simulink model "SingleEcho"  (R2024a)
settings: Solver=VariableStepAuto  StartTime=0  StopTime=inf  RelTol=1e-3
libraries: dspsrcs4 x2, audiosources x1, dspsnks4 x1
settings Model: Creator=johannesarizie  LastModifiedBy=johannesarizie

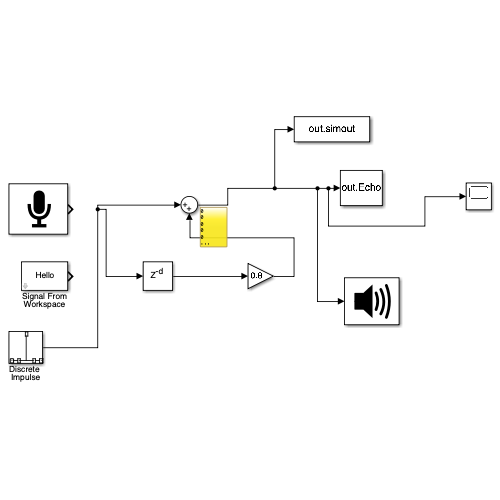
[thumbnail: Simulink's stored preview of the top-level diagram]
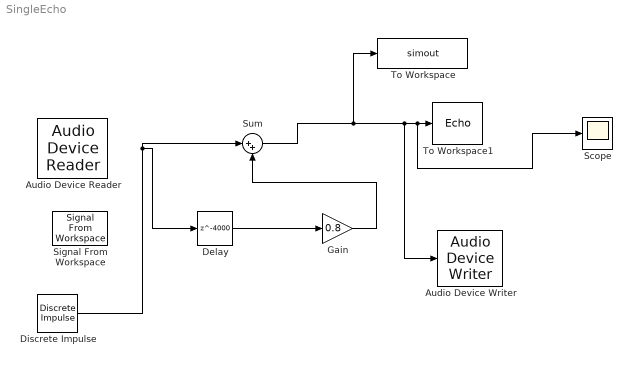
== system SingleEcho ==
  Audio Device Reader : audiosources/Audio Device Reader  Driver=CoreAudio  Device=Default  SampleRate=44100  NumChannels=1  SamplesPerFrame=1024  BitDepth=16-bit integer  NumBuffers=10  DefaultInputChannelMapping=on  InputChannelMapping=1:2  OutputNumOverrunSamples=off  OutputDataType=double  DriverIdx=5  DeviceWarnFlag=''
  Audio Device Writer : dspsnks4/Audio Device Writer  Driver=CoreAudio  Device=Default  InheritSampleRate=on  SampleRate=44100  BitDepth=16-bit integer  BufferSize=4096  NumBuffers=10  DefaultOutputChannelMapping=on  OutputChannelMapping=1:2  OutputNumUnderrunSamples=off  DriverIdx=5  DeviceWarnFlag=''
  Delay : Delay  DelayLength=4000  InitialCondition=0
  Discrete Impulse : dspsrcs4/Discrete  Impulse  Delay=0  SampleTime=1/8000  FrameSample=64  OutputFrames=off  dataType=Inherit via back propagation  isSigned=on  wordLen=16  udDataType=sfix(16)  fracBitsMode=Best precision  numFracBits=15  OutDataTypeStr=Inherit: Inherit via back propagation  LastOutDataTypeStr=Inherit: Inherit via back propagation
  Gain : Gain  Gain=0.8
  Scope : Scope
  Signal From Workspace : dspsrcs4/Signal From Workspace  X=Hello  Ts=1/8000  nsamps=64  OutputAfterFinalValue=Cyclic repetition  ignoreOrWarnInputAndFrameLengths=off  OutputFrames=off
  Sum : Sum  Inputs=|++
  To Workspace : ToWorkspace  VariableName=simout  SaveFormat=Timeseries  SampleTime=-1
      settings: Save2DSignal=2-D array (concatenate along first dimension)
  To Workspace1 : ToWorkspace  VariableName=Echo  SampleTime=-1
      settings: Save2DSignal=2-D array (concatenate along first dimension)
  wires:
  Delay/1 -> Gain/1
  Gain/1 -> Sum/2
  Sum/1 -> Audio Device Writer/1, Scope/1, To Workspace1/1, To Workspace/1
  Discrete Impulse/1 -> Sum/1, Delay/1
